simulink model "updated_reqtable"  (R2022b)
settings: Solver=VariableStepAuto  StartTime=0.0  StopTime=10.0  RelTol=1e-3
settings Model: Creator=16479  LastModifiedBy=16479

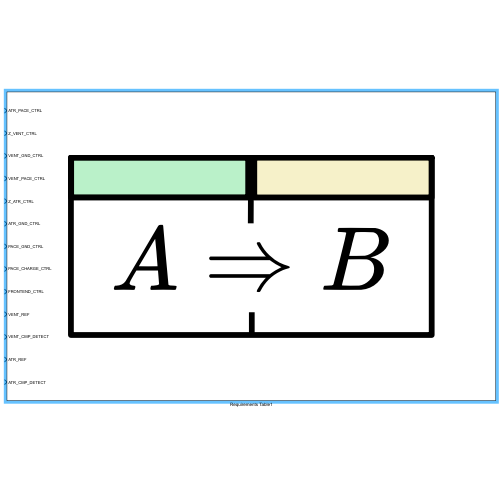
[thumbnail: Simulink's stored preview of the top-level diagram]
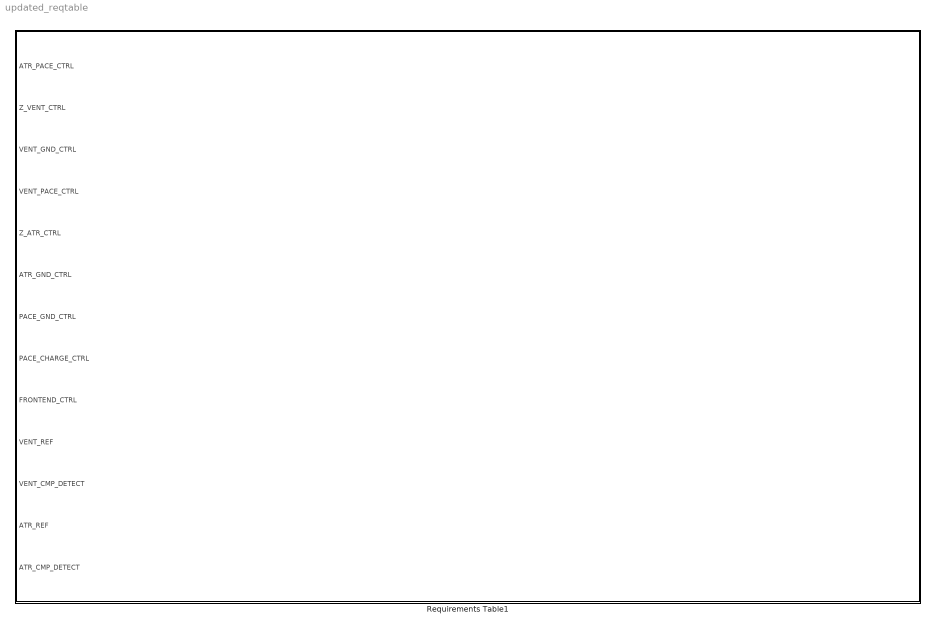
== system updated_reqtable ==
  Requirements Table1 : Requirements Table  TreatAsAtomicUnit=on

== stateflow chart updated_reqtable/Requirements Table1 ==
  (default) -> (junction 1073759175)
  (junction 1073759175) -> (junction 1073759176) : {
      | % SF_REQ_REV_07
      | }
  (junction 1073759176) -> (junction 1073759178) : {
      | % HEADER_ASSIGNMENTS
      |
      | }
  (junction 1073759178) -> (junction 1073759180) : {
      | % START_A_4
      | }
  (junction 1073759180) -> (junction 1073759182) : {
      | }
  (junction 1073759182) -> (junction 1073759184)
  (junction 1073759184) -> (junction 1073759186) : {
      | }
  (junction 1073759186) -> (junction 1073759188) : {
      | % END_A_4
      | }
  (junction 1073759188) -> (junction 1073759190) : {
      | % START_R_73
      | }
  (junction 1073759190) -> (junction 1073759192) : {
      | }
  (junction 1073759192) -> (junction 1073759194)
  (junction 1073759194) -> (junction 1073759196) [order 1] : [(VENT_PACE_CTRL == false) && (ATR_PACE_CTRL == false) && (VENT_GND_CTRL == false) && (ATR_PACE_CTRL == false) && (PACE_GND_CTRL == false) && (PACE_CHARGE_CTRL == false) && (FRONTEND_CTL == false) && (VENT_CMP_REF_PWM == 0) && (ATR_CMP_REF_PWM == 0) && (PACING_REF_PWM == 0) && (Z_ATR_CTRL == false) && (Z_VENT_CTRL == false)]
  (junction 1073759194) -> (junction 1073759202) [order 2]
  (junction 1073759196) -> (junction 1073759198) : {
      |
      |
      |
      |
      |
      |
      |
      |
      |
      |
      |
      |
      |
      | }
  (junction 1073759198) -> (junction 1073759200) : {
      | }
  (junction 1073759200) -> (junction 1073759202)
  (junction 1073759202) -> (junction 1073759204)
  (junction 1073759204) -> (junction 1073759206) : {
      | % END_R_73
      | }
  (junction 1073759206) -> (junction 1073759208) : {
      | % START_R_16
      | }
  (junction 1073759208) -> (junction 1073759210) : {
      | }
  (junction 1073759210) -> (junction 1073759212) : {
      |
      |
      |
      |
      |
      |
      |
      |
      |
      |
      |
      |
      |
      | }
  (junction 1073759212) -> (junction 1073759214) : {
      | }
  (junction 1073759214) -> (junction 1073759216) : {
      | % START_R_79
      | }
  (junction 1073759216) -> (junction 1073759218) : {
      | }
  (junction 1073759218) -> (junction 1073759220)
  (junction 1073759220) -> (junction 1073759222) [order 1] : [(Mode == 1)]
  (junction 1073759220) -> (junction 1073759228) [order 2]
  (junction 1073759222) -> (junction 1073759224) : {
      |
      |
      |
      |
      |
      |
      |
      |
      |
      |
      |
      |
      |
      | }
  (junction 1073759224) -> (junction 1073759226) : {
      | }
  (junction 1073759226) -> (junction 1073759228)
  (junction 1073759228) -> (junction 1073759230)
  (junction 1073759230) -> (junction 1073759232) : {
      | % END_R_79
      | }
  (junction 1073759232) -> (junction 1073759234) : {
      | % START_R_19
      | }
  (junction 1073759234) -> (junction 1073759236) : {
      | }
  (junction 1073759236) -> (junction 1073759238)
  (junction 1073759238) -> (junction 1073759240) [order 1] : [duration((VENT_PACE_CTRL == false) && (PACE_CHARGE_CTRL== true) && (VENT_GND_CTRL == true) && (PACE_GND_CTRL == true) && (Z_VENT_CTRL == false)) >= 60000/LRL-VPW]
  (junction 1073759238) -> (junction 1073759246) [order 2]
  (junction 1073759240) -> (junction 1073759242) : {
      | VENT_PACE_CTRL == true
      |
      | PACE_CHARGE_CTRL == false
      |
      | VENT_GND_CTRL == false
      | PACE_GND_CTRL == true
      |
      | Z_VENT_CTRL == false
      |
      |
      |
      |
      |
      | }
  (junction 1073759242) -> (junction 1073759244) : {
      | }
  (junction 1073759244) -> (junction 1073759246)
  (junction 1073759246) -> (junction 1073759248)
  (junction 1073759248) -> (junction 1073759250) : {
      | % END_R_19
      | }
  (junction 1073759250) -> (junction 1073759252) : {
      | % START_R_22
      | }
  (junction 1073759252) -> (junction 1073759254) : {
      | }
  (junction 1073759254) -> (junction 1073759256)
  (junction 1073759256) -> (junction 1073759258) [order 1] : [duration((VENT_PACE_CTRL == true) && (PACE_CHARGE_CTRL == false) && (VENT_GND_CTRL == false) && (PACE_GND_CTRL == true) && (Z_VENT_CTRL == false)) >= VPW]
  (junction 1073759256) -> (junction 1073759264) [order 2]
  (junction 1073759258) -> (junction 1073759260) : {
      | VENT_PACE_CTRL == false
      |
      | PACE_CHARGE_CTRL == true
      |
      | VENT_GND_CTRL == true
      | PACE_GND_CTRL == true
      |
      | Z_VENT_CTRL == false
      |
      |
      |
      |
      |
      | }
  (junction 1073759260) -> (junction 1073759262) : {
      | }
  (junction 1073759262) -> (junction 1073759264)
  (junction 1073759264) -> (junction 1073759266)
  (junction 1073759266) -> (junction 1073759268) : {
      | % END_R_22
      | }
  (junction 1073759268) -> (junction 1073759270) : {
      | % START_R_76
      | }
  (junction 1073759270) -> (junction 1073759272) : {
      | }
  (junction 1073759272) -> (junction 1073759274)
  (junction 1073759274) -> (junction 1073759276) [order 1] : [(Mode ~=1)]
  (junction 1073759274) -> (junction 1073759282) [order 2]
  (junction 1073759276) -> (junction 1073759278) : {
      | VENT_PACE_CTRL == false
      | ATR_PACE_CTRL == false
      | VENT_GND_CTRL == false
      | ATR_PACE_CTRL == false
      | PACE_GND_CTRL == false
      | PACE_CHARGE_CTRL == false
      | FRONTEND_CTL == false
      | VENT_CMP_REF_PWM == 0
      | ATR_CMP_REF_PWM == 0
      | PACING_REF_PWM == 0
      | Z_ATR_CTRL == false
      | Z_VENT_CTRL == false
      |
      | }
  (junction 1073759278) -> (junction 1073759280) : {
      | }
  (junction 1073759280) -> (junction 1073759282)
  (junction 1073759282) -> (junction 1073759284)
  (junction 1073759284) -> (junction 1073759286) : {
      | % END_R_76
      | }
  (junction 1073759286) -> (junction 1073759288) : {
      | % END_R_16
      | }
  (junction 1073759288) -> (junction 1073759746) : {
      | % START_R_1
      | }
  (junction 1073759746) -> (junction 1073759748) : {
      | }
  (junction 1073759748) -> (junction 1073759750) : {
      |
      |
      |
      |
      |
      |
      |
      |
      |
      |
      |
      |
      |
      | }
  (junction 1073759750) -> (junction 1073759752) : {
      | }
  (junction 1073759752) -> (junction 1073759754) : {
      | % START_R_10
      | }
  (junction 1073759754) -> (junction 1073759756) : {
      | }
  (junction 1073759756) -> (junction 1073759758)
  (junction 1073759758) -> (junction 1073759760) [order 1] : [duration((ATR_PACE_CTRL == false) && (PACE_CHARGE_CTRL == true) && (PACE_GND_CTRL == true) && (ATR_GND_CTRL == true) && (Z_ATR_CTRL == false)) >= 60000/LRL-APW]
  (junction 1073759758) -> (junction 1073759766) [order 2]
  (junction 1073759760) -> (junction 1073759762) : {
      | ATR_PACE_CTRL == true
      |
      | PACE_CHARGE_CTRL == false
      |
      | PACE_GND_CTRL == true
      | ATR_GND_CTRL == false
      |
      | Z_ATR_CTRL == false
      |
      |
      |
      |
      |
      | }
  (junction 1073759762) -> (junction 1073759764) : {
      | }
  (junction 1073759764) -> (junction 1073759766)
  (junction 1073759766) -> (junction 1073759768)
  (junction 1073759768) -> (junction 1073759770) : {
      | % END_R_10
      | }
  (junction 1073759770) -> (junction 1073759772) : {
      | % START_R_13
      | }
  (junction 1073759772) -> (junction 1073759774) : {
      | }
  (junction 1073759774) -> (junction 1073759776)
  (junction 1073759776) -> (junction 1073759778) [order 1] : [duration((ATR_PACE_CTRL == true) && (PACE_CHARGE_CTRL == false) && (PACE_GND_CTRL == true) && (ATR_GND_CTRL == false) && (Z_ATR_CTRL == false)) >= APW]
  (junction 1073759776) -> (junction 1073759784) [order 2]
  (junction 1073759778) -> (junction 1073759780) : {
      | ATR_PACE_CTRL == false
      |
      | PACE_CHARGE_CTRL == true
      |
      | PACE_GND_CTRL == true
      | ATR_GND_CTRL == true
      |
      | Z_ATR_CTRL == false
      |
      |
      |
      |
      |
      | }
  (junction 1073759780) -> (junction 1073759782) : {
      | }
  (junction 1073759782) -> (junction 1073759784)
  (junction 1073759784) -> (junction 1073759786)
  (junction 1073759786) -> (junction 1073759808) : {
      | % END_R_13
      | }
  (junction 1073759808) -> (junction 1073759837) : {
      | % START_R_91
      | }
  (junction 1073759837) -> (junction 1073759839) : {
      | }
  (junction 1073759839) -> (junction 1073759841)
  (junction 1073759841) -> (junction 1073759843) [order 1] : [(Mode == 2)]
  (junction 1073759841) -> (junction 1073759849) [order 2]
  (junction 1073759843) -> (junction 1073759845) : {
      |
      |
      |
      |
      |
      |
      |
      |
      |
      |
      |
      |
      |
      | }
  (junction 1073759845) -> (junction 1073759847) : {
      | }
  (junction 1073759847) -> (junction 1073759849)
  (junction 1073759849) -> (junction 1073759851)
  (junction 1073759851) -> (junction 1073759853) : {
      | % END_R_91
      | }
  (junction 1073759853) -> (junction 1073759816) : {
      | % START_R_88
      | }
  (junction 1073759816) -> (junction 1073759818) : {
      | }
  (junction 1073759818) -> (junction 1073759820)
  (junction 1073759820) -> (junction 1073759822) [order 1] : [(Mode ~=2)]
  (junction 1073759820) -> (junction 1073759828) [order 2]
  (junction 1073759822) -> (junction 1073759824) : {
      | VENT_PACE_CTRL == false
      | ATR_PACE_CTRL == false
      | VENT_GND_CTRL == false
      | ATR_PACE_CTRL == false
      | PACE_GND_CTRL == false
      | PACE_CHARGE_CTRL == false
      | FRONTEND_CTL == false
      | VENT_CMP_REF_PWM == 0
      | ATR_CMP_REF_PWM == 0
      | PACING_REF_PWM == 0
      | Z_ATR_CTRL == false
      | Z_VENT_CTRL == false
      |
      | }
  (junction 1073759824) -> (junction 1073759826) : {
      | }
  (junction 1073759826) -> (junction 1073759828)
  (junction 1073759828) -> (junction 1073759830)
  (junction 1073759830) -> (junction 1073759832) : {
      | % END_R_88
      | }
  (junction 1073759832) -> (junction 1073759810) : {
      | % END_R_1
      | }
  (junction 1073759810) -> (junction 1073760241) : {
      | % START_R_25
      | }
  (junction 1073760241) -> (junction 1073760243) : {
      | }
  (junction 1073760243) -> (junction 1073760245) : {
      |
      |
      |
      |
      |
      |
      |
      |
      |
      |
      |
      |
      |
      | }
  (junction 1073760245) -> (junction 1073760247) : {
      | }
  (junction 1073760247) -> (junction 1073760249) : {
      | % START_R_97
      | }
  (junction 1073760249) -> (junction 1073760251) : {
      | }
  (junction 1073760251) -> (junction 1073760253)
  (junction 1073760253) -> (junction 1073760255) [order 1] : [(Mode == 3)]
  (junction 1073760253) -> (junction 1073760261) [order 2]
  (junction 1073760255) -> (junction 1073760257) : {
      |
      |
      |
      |
      |
      |
      |
      |
      |
      |
      |
      |
      |
      | }
  (junction 1073760257) -> (junction 1073760259) : {
      | }
  (junction 1073760259) -> (junction 1073760261)
  (junction 1073760261) -> (junction 1073760263)
  (junction 1073760263) -> (junction 1073760265) : {
      | % END_R_97
      | }
  (junction 1073760265) -> (junction 1073760405) : {
      | % START_R_100
      | }
  (junction 1073760405) -> (junction 1073760407) : {
      | }
  (junction 1073760407) -> (junction 1073760409)
  (junction 1073760409) -> (junction 1073760411) [order 1] : [(Mode ~=3)]
  (junction 1073760409) -> (junction 1073760417) [order 2]
  (junction 1073760411) -> (junction 1073760413) : {
      | VENT_PACE_CTRL == false
      | ATR_PACE_CTRL == false
      | VENT_GND_CTRL == false
      | ATR_PACE_CTRL == false
      | PACE_GND_CTRL == false
      | PACE_CHARGE_CTRL == false
      | FRONTEND_CTL == false
      | VENT_CMP_REF_PWM == 0
      | ATR_CMP_REF_PWM == 0
      | PACING_REF_PWM == 0
      | Z_ATR_CTRL == false
      | Z_VENT_CTRL == false
      |
      | }
  (junction 1073760413) -> (junction 1073760415) : {
      | }
  (junction 1073760415) -> (junction 1073760417)
  (junction 1073760417) -> (junction 1073760419)
  (junction 1073760419) -> (junction 1073760421) : {
      | % END_R_100
      | }
  (junction 1073760421) -> (junction 1073760958) : {
      | % START_R_28
      | }
  (junction 1073760958) -> (junction 1073760960) : {
      | }
  (junction 1073760960) -> (junction 1073760962)
  (junction 1073760962) -> (junction 1073760964) [order 1] : [(FRONTEND_CTRL == true ) && (VENT_PACE_CTRL== false) && (PACE_CHARGE_CTRL == true) && (PACE_GND_CTRL == true) && (VENT_GND_CTRL == true) && (Z_VENT_CTRL == false)]
  (junction 1073760962) -> (junction 1073760970) [order 2]
  (junction 1073760964) -> (junction 1073760966) : {
      |
      |
      |
      |
      |
      |
      |
      |
      |
      |
      |
      |
      |
      | }
  (junction 1073760966) -> (junction 1073760968) : {
      | }
  (junction 1073760968) -> (junction 1073760970)
  (junction 1073760970) -> (junction 1073760972)
  (junction 1073760972) -> (junction 1073760974) : {
      | % END_R_28
      | }
  (junction 1073760974) -> (junction 1073760321) : {
      | % START_R_31
      | }
  (junction 1073760321) -> (junction 1073760323) : {
      | }
  (junction 1073760323) -> (junction 1073760325)
  (junction 1073760325) -> (junction 1073760327) [order 1] : [duration((FRONTEND_CTRL == true ) && (VENT_PACE_CTRL == true) && (PACE_CHARGE_CTRL == false) && (PACE_GND_CTRL == true) && (VENT_GND_CTRL == false) && (Z_VENT_CTRL == false)) >= VPW]
  (junction 1073760325) -> (junction 1073760369) [order 2]
  (junction 1073760327) -> (junction 1073760329) : {
      |
      |
      |
      |
      |
      |
      |
      |
      |
      |
      |
      |
      |
      | }
  (junction 1073760329) -> (junction 1073760331) : {
      | }
  (junction 1073760331) -> (junction 1073760333) : {
      | % START_R_55
      | }
  (junction 1073760333) -> (junction 1073760335) : {
      | }
  (junction 1073760335) -> (junction 1073760337)
  (junction 1073760337) -> (junction 1073760339) [order 1] : [(VENT_CMP_DETECT == true)]
  (junction 1073760337) -> (junction 1073760345) [order 2]
  (junction 1073760339) -> (junction 1073760341) : {
      |
      | (FRONTEND_CTRL) == false
      | (PACE_CHARGE_CTRL) == true
      | (VENT_PACE_CTRL) == false
      |
      | (PACE_GND_CTRL) == true
      | (VENT_GND_CTRL) == true
      | (Z_VENT_CTRL) == false
      |
      |
      |
      |
      |
      | }
  (junction 1073760341) -> (junction 1073760343) : {
      | }
  (junction 1073760343) -> (junction 1073760345)
  (junction 1073760345) -> (junction 1073760347)
  (junction 1073760347) -> (junction 1073760349) : {
      | % END_R_55
      | }
  (junction 1073760349) -> (junction 1073760351) : {
      | % START_R_58
      | }
  (junction 1073760351) -> (junction 1073760353) : {
      | }
  (junction 1073760353) -> (junction 1073760355)
  (junction 1073760355) -> (junction 1073760357) [order 1] : [(VENT_CMP_DETECT== false)]
  (junction 1073760355) -> (junction 1073760363) [order 2]
  (junction 1073760357) -> (junction 1073760359) : {
      |
      | (FRONTEND_CTRL) == true
      | (PACE_CHARGE_CTRL) == true
      | (VENT_PACE_CTRL) == false
      |
      | (PACE_GND_CTRL) == true
      | (VENT_GND_CTRL) == true
      | (Z_VENT_CTRL) == false
      |
      |
      |
      |
      |
      | }
  (junction 1073760359) -> (junction 1073760361) : {
      | }
  (junction 1073760361) -> (junction 1073760363)
  (junction 1073760363) -> (junction 1073760365)
  (junction 1073760365) -> (junction 1073760367) : {
      | % END_R_58
      | }
  (junction 1073760367) -> (junction 1073760369)
  (junction 1073760369) -> (junction 1073760371)
  (junction 1073760371) -> (junction 1073760373) : {
      | % END_R_31
      | }
  (junction 1073760373) -> (junction 1073760375) : {
      | % START_R_34
      | }
  (junction 1073760375) -> (junction 1073760377) : {
      | }
  (junction 1073760377) -> (junction 1073760379)
  (junction 1073760379) -> (junction 1073760381) [order 1] : [(FRONTEND_CTRL == false) && (VENT_PACE_CTRL == false) && (PACE_CHARGE_CTRL == true) && (PACE_GND_CTRL == true) && (VENT_GND_CTRL == true) && (Z_VENT_CTRL== false)]
  (junction 1073760379) -> (junction 1073760387) [order 2]
  (junction 1073760381) -> (junction 1073760383) : {
      |
      | (FRONTEND_CTRL) == true
      | (PACE_CHARGE_CTRL) == true
      | (VENT_PACE_CTRL) == false
      |
      | (PACE_GND_CTRL) == true
      | (VENT_GND_CTRL) == true
      | (Z_VENT_CTRL) == false
      |
      |
      |
      |
      |
      | }
  (junction 1073760383) -> (junction 1073760385) : {
      | }
  (junction 1073760385) -> (junction 1073760387)
  (junction 1073760387) -> (junction 1073760389)
  (junction 1073760389) -> (junction 1073760391) : {
      | % END_R_34
      | }
  (junction 1073760391) -> (junction 1073760393) : {
      | % END_R_25
      | }
  (junction 1073760393) -> (junction 1073760632) : {
      | % START_R_37
      | }
  (junction 1073760632) -> (junction 1073760634) : {
      | }
  (junction 1073760634) -> (junction 1073760636) : {
      |
      |
      |
      |
      |
      |
      |
      |
      |
      |
      |
      |
      |
      | }
  (junction 1073760636) -> (junction 1073760638) : {
      | }
  (junction 1073760638) -> (junction 1073760640) : {
      | % START_R_103
      | }
  (junction 1073760640) -> (junction 1073760642) : {
      | }
  (junction 1073760642) -> (junction 1073760644)
  (junction 1073760644) -> (junction 1073760646) [order 1] : [(Mode == 4)]
  (junction 1073760644) -> (junction 1073760652) [order 2]
  (junction 1073760646) -> (junction 1073760648) : {
      |
      |
      |
      |
      |
      |
      |
      |
      |
      |
      |
      |
      |
      | }
  (junction 1073760648) -> (junction 1073760650) : {
      | }
  (junction 1073760650) -> (junction 1073760652)
  (junction 1073760652) -> (junction 1073760654)
  (junction 1073760654) -> (junction 1073760656) : {
      | % END_R_103
      | }
  (junction 1073760656) -> (junction 1073760796) : {
      | % START_R_106
      | }
  (junction 1073760796) -> (junction 1073760798) : {
      | }
  (junction 1073760798) -> (junction 1073760800)
  (junction 1073760800) -> (junction 1073760802) [order 1] : [(Mode ~=4)]
  (junction 1073760800) -> (junction 1073760808) [order 2]
  (junction 1073760802) -> (junction 1073760804) : {
      | VENT_PACE_CTRL == false
      | ATR_PACE_CTRL == false
      | VENT_GND_CTRL == false
      | ATR_PACE_CTRL == false
      | PACE_GND_CTRL == false
      | PACE_CHARGE_CTRL == false
      | FRONTEND_CTL == false
      | VENT_CMP_REF_PWM == 0
      | ATR_CMP_REF_PWM == 0
      | PACING_REF_PWM == 0
      | Z_ATR_CTRL == false
      | Z_VENT_CTRL == false
      |
      | }
  (junction 1073760804) -> (junction 1073760806) : {
      | }
  (junction 1073760806) -> (junction 1073760808)
  (junction 1073760808) -> (junction 1073760810)
  (junction 1073760810) -> (junction 1073760812) : {
      | % END_R_106
      | }
  (junction 1073760812) -> (junction 1073760937) : {
      | % START_R_40
      | }
  (junction 1073760937) -> (junction 1073760939) : {
      | }
  (junction 1073760939) -> (junction 1073760941)
  (junction 1073760941) -> (junction 1073760943) [order 1] : [(FRONTEND_CTRL == true ) && (ATR_PACE_CTRL == false) && (PACE_CHARGE_CTRL == true) && (PACE_GND_CTRL== true) && (ATR_GND_CTRL == true) && (Z_ATR_CTRL == false)]
  (junction 1073760941) -> (junction 1073760949) [order 2]
  (junction 1073760943) -> (junction 1073760945) : {
      |
      |
      |
      |
      |
      |
      |
      |
      |
      |
      |
      |
      |
      | }
  (junction 1073760945) -> (junction 1073760947) : {
      | }
  (junction 1073760947) -> (junction 1073760949)
  (junction 1073760949) -> (junction 1073760951)
  (junction 1073760951) -> (junction 1073760953) : {
      | % END_R_40
      | }
  (junction 1073760953) -> (junction 1073760878) : {
      | % START_R_43
      | }
  (junction 1073760878) -> (junction 1073760880) : {
      | }
  (junction 1073760880) -> (junction 1073760882)
  (junction 1073760882) -> (junction 1073760884) [order 1] : [duration((FRONTEND_CTRL== true ) && (ATR_PACE_CTRL == true) && (PACE_CHARGE_CTRL == false) && (PACE_GND_CTRL == true) && (ATR_GND_CTRL == false) && (Z_ATR_CTRL == false)) >= APW]
  (junction 1073760882) -> (junction 1073760926) [order 2]
  (junction 1073760884) -> (junction 1073760886) : {
      |
      |
      |
      |
      |
      |
      |
      |
      |
      |
      |
      |
      |
      | }
  (junction 1073760886) -> (junction 1073760888) : {
      | }
  (junction 1073760888) -> (junction 1073760890) : {
      | % START_R_67
      | }
  (junction 1073760890) -> (junction 1073760892) : {
      | }
  (junction 1073760892) -> (junction 1073760894)
  (junction 1073760894) -> (junction 1073760896) [order 1] : [(ATR_CMP_DETECT == true)]
  (junction 1073760894) -> (junction 1073760902) [order 2]
  (junction 1073760896) -> (junction 1073760898) : {
      |
      | (FRONTEND_CTRL) == false
      | (PACE_CHARGE_CTRL) == true
      | (ATR_PACE_CTRL) == false
      |
      | (PACE_GND_CTRL) == true
      | (ATR_GND_CTRL) == true
      | (Z_ATR_CTRL) == false
      |
      |
      |
      |
      |
      | }
  (junction 1073760898) -> (junction 1073760900) : {
      | }
  (junction 1073760900) -> (junction 1073760902)
  (junction 1073760902) -> (junction 1073760904)
  (junction 1073760904) -> (junction 1073760906) : {
      | % END_R_67
      | }
  (junction 1073760906) -> (junction 1073760908) : {
      | % START_R_70
      | }
  (junction 1073760908) -> (junction 1073760910) : {
      | }
  (junction 1073760910) -> (junction 1073760912)
  (junction 1073760912) -> (junction 1073760914) [order 1] : [(ATR_CMP_DETECT == false)]
  (junction 1073760912) -> (junction 1073760920) [order 2]
  (junction 1073760914) -> (junction 1073760916) : {
      |
      | (FRONTEND_CTRL) == true
      | (PACE_CHARGE_CTRL) == true
      | (ATR_PACE_CTRL) == false
      |
      | (PACE_GND_CTRL) == true
      | (ATR_GND_CTRL) == true
      | (Z_ATR_CTRL) == false
      |
      |
      |
      |
      |
      | }
  (junction 1073760916) -> (junction 1073760918) : {
      | }
  (junction 1073760918) -> (junction 1073760920)
  (junction 1073760920) -> (junction 1073760922)
  (junction 1073760922) -> (junction 1073760924) : {
      | % END_R_70
      | }
  (junction 1073760924) -> (junction 1073760926)
  (junction 1073760926) -> (junction 1073760928)
  (junction 1073760928) -> (junction 1073760987) : {
      | % END_R_43
      | }
  (junction 1073760987) -> (junction 1073760766) : {
      | % START_R_46
      | }
  (junction 1073760766) -> (junction 1073760768) : {
      | }
  (junction 1073760768) -> (junction 1073760770)
  (junction 1073760770) -> (junction 1073760772) [order 1] : [(FRONTEND_CTRL == false) && (ATR_PACE_CTRL == false) && (PACE_CHARGE_CTRL == true) && (PACE_GND_CTRL == true) && (ATR_GND_CTRL == true) && (Z_ATR_CTRL == false)]
  (junction 1073760770) -> (junction 1073760778) [order 2]
  (junction 1073760772) -> (junction 1073760774) : {
      |
      | (FRONTEND_CTRL) == true
      | (PACE_CHARGE_CTRL) == true
      | (ATR_PACE_CTRL) == false
      |
      | (PACE_GND_CTRL) == true
      | (ATR_GND_CTRL) == true
      | (Z_ATR_CTRL) == false
      |
      |
      |
      |
      |
      | }
  (junction 1073760774) -> (junction 1073760776) : {
      | }
  (junction 1073760776) -> (junction 1073760778)
  (junction 1073760778) -> (junction 1073760780)
  (junction 1073760780) -> (junction 1073760782) : {
      | % END_R_46
      | }
  (junction 1073760782) -> (junction 1073760784) : {
      | % END_R_37
      | }
  data: ATR_PACE_CTRL input boolean; Z_VENT_CTRL input boolean; VENT_GND_CTRL input boolean; VENT_PACE_CTRL input boolean; Z_ATR_CTRL input boolean; ATR_GND_CTRL input boolean; PACE_GND_CTRL input boolean; PACE_CHARGE_CTRL input boolean; FRONTEND_CTRL input boolean; VENT_REF input int8; VENT_CMP_DETECT input boolean; ATR_REF input int8; LRL constant int8; VENT_PULSE_WIDTH constant int8; ATR_PULSE_WIDTH constant int8; ATR_CMP_DETECT input boolean
